simulink model "Parcial_2"  (R2020a)
settings: Solver=VariableStepAuto  StartTime=0.0  StopTime=5  RelTol=1e-3
settings Model: Creator=oscarvch03  LastModifiedBy=oscarvch03

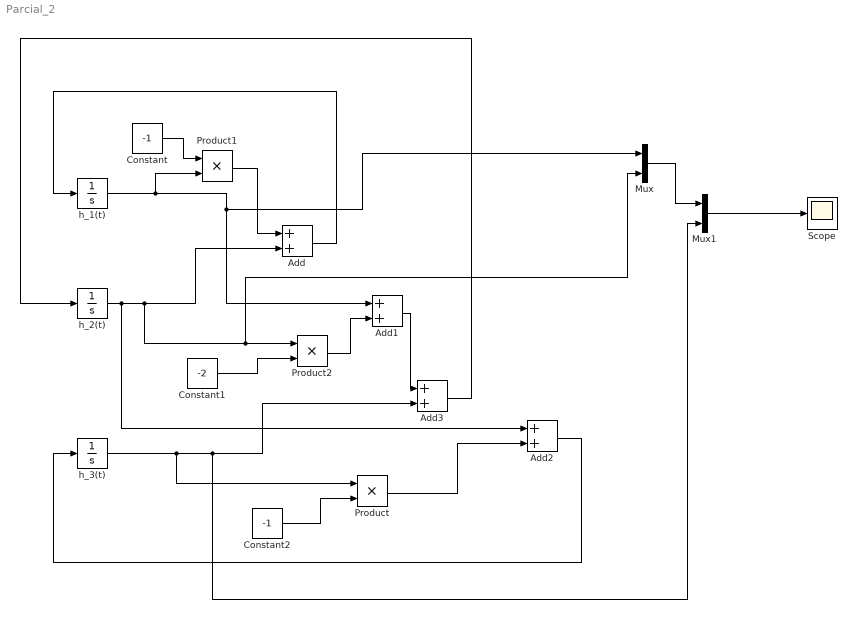
== system Parcial_2 ==
  Add{,1..3} (4 alike) : Sum
  Constant : Constant  Value=-1
  Constant1 : Constant  Value=-2
  Constant2 : Constant  Value=-1
  Mux : Mux  Inputs=2
  Mux1 : Mux  Inputs=2
  Product : Product
  Product1 : Product
  Product2 : Product
  Scope : Scope
  h_1(t) : Integrator  InitialCondition=0.2
  h_2(t) : Integrator  InitialCondition=0.2
  h_3(t) : Integrator  InitialCondition=0.1
  wires:
  h_1(t)/1 -> Mux/1, Add1/1, Product1/2
  Constant/1 -> Product1/1
  h_2(t)/1 -> Add2/1, Mux/2, Product2/1, Add/2
  Product1/1 -> Add/1
  Add/1 -> h_1(t)/1
  Constant1/1 -> Product2/2
  Product2/1 -> Add1/2
  h_3(t)/1 -> Add3/2, Mux1/2, Product/1
  Add1/1 -> Add3/1
  Add3/1 -> h_2(t)/1
  Constant2/1 -> Product/2
  Product/1 -> Add2/2
  Add2/1 -> h_3(t)/1
  Mux/1 -> Mux1/1
  Mux1/1 -> Scope/1
